simulink model "MotorMBD_TOP"  (R2018b)
settings: Solver=VariableStepAuto  StartTime=0.0  StopTime=1  RelTol=1e-3
values from neighbouring files (symbols this model uses):
  Jm = 0.0001    [parameter.m]
  Kdi = Ra*wc    (= 1002.79637503)    [parameter.m]
  Kdp = Ld*wc    (= 0.913156264643)    [parameter.m]
  Kqi = Ra*wc    (= 1002.79637503)    [parameter.m]
  Kqp = Lq*wc    (= 0.996932068739)    [parameter.m]
  Ksa = 3/Ksp    (= 35.8098621957)    [parameter.m]
  Ksi = Jm*wsc*(wsc/5)    (= 14.0367707038)    [parameter.m]
  Ksp = Jm*wsc    (= 0.0837758040957)    [parameter.m]
  Ld = 1.09e-4    (= 0.000109)    [parameter.m]
  Lq = 1.19e-4    (= 0.000119)    [parameter.m]
  Phia = 4.5e-3    (= 0.0045)    [parameter.m]
  Pn = 4    [parameter.m]
  Ra = 0.1197    [parameter.m]
  rpm2wrm = (2*pi)/60    (= 0.10471975512)    [parameter.m]
  taul = 0    [parameter.m]
  wrm2rpm = 60/(2*pi)    (= 9.54929658551)    [parameter.m]
settings Model: Creator=81803  LastModifiedBy=81803

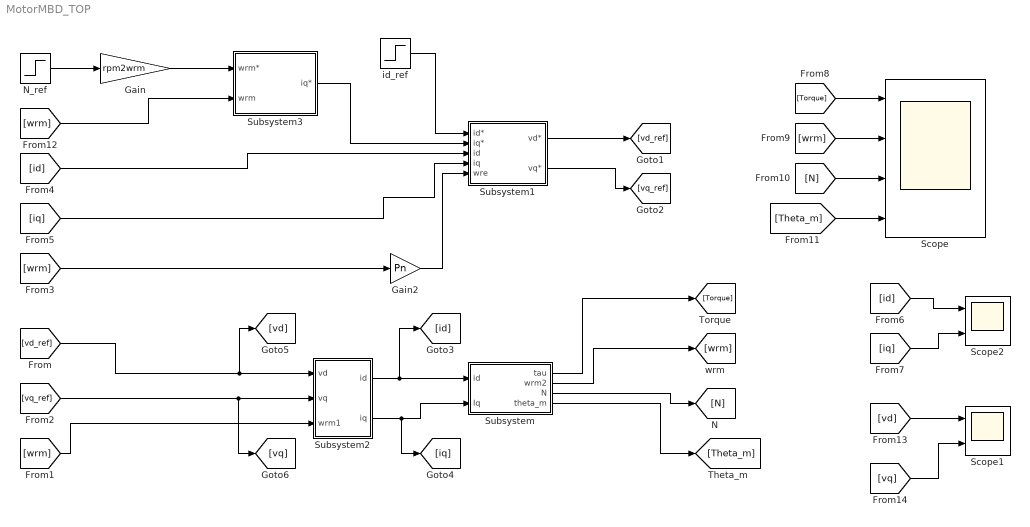
== system MotorMBD_TOP ==
  Gain : Gain  Gain=rpm2wrm
  Gain2 : Gain  Gain=Pn
  N_ref : Step  Time=0  After=3000  SampleTime=0
  Scope : Scope  NumInputPorts=4
  Scope1 : Scope  NumInputPorts=2
  Scope2 : Scope  NumInputPorts=2
  Subsystem : Subsystem
  Subsystem1 : Subsystem
  Subsystem2 : Subsystem
  Subsystem3 : Subsystem
  id_ref : Step  Time=0  After=0  SampleTime=0
  wires:
  id_ref/1 -> Subsystem1/1(id*)
  Subsystem3/1(iq*) -> Subsystem1/2(iq*)
  [id] -> Subsystem1/3(id)
  [iq] -> Subsystem1/4(iq)
  [wrm] -> Gain2/1
  Subsystem1/1(vd*) -> [vd_ref]
  Subsystem1/2(vq*) -> [vq_ref]
  [vd_ref] -> [vd], Subsystem2/1(vd)
  Subsystem2/1(id) -> [id], Subsystem/1(id)
  [vq_ref] -> [vq], Subsystem2/2(vq)
  Subsystem2/2(iq) -> [iq], Subsystem/2(Iq)
  Subsystem/1(tau) -> [Torque]
  [wrm] -> Subsystem2/3(wrm1)
  Subsystem/4(theta_m) -> [Theta_m]
  Subsystem/2(wrm2) -> [wrm]
  Subsystem/3(N) -> [N]
  [id] -> Scope2/1
  [iq] -> Scope2/2
  [Torque] -> Scope/1
  [wrm] -> Scope/2
  [N] -> Scope/3
  [Theta_m] -> Scope/4
  Gain/1 -> Subsystem3/1(wrm*)
  [wrm] -> Subsystem3/2(wrm)
  N_ref/1 -> Gain/1
  Gain2/1 -> Subsystem1/5(wre)
  [vd] -> Scope1/1
  [vq] -> Scope1/2

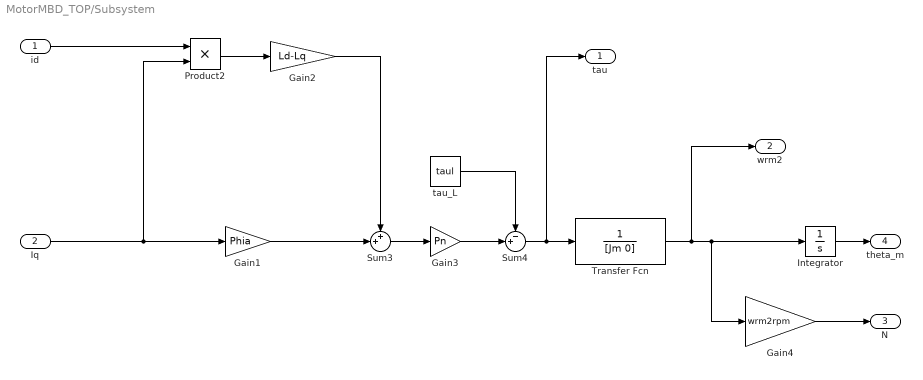
== system MotorMBD_TOP/Subsystem ==
  id : Inport
  Iq : Inport  Port=2
  Gain1 : Gain  Gain=Phia
  Gain2 : Gain  Gain=Ld-Lq
  Gain3 : Gain  Gain=Pn
  Gain4 : Gain  Gain=wrm2rpm
  Integrator : Integrator
  Product2 : Product
  Sum3 : Sum  Inputs=++|
  Sum4 : Sum  Inputs=-+|
  Transfer Fcn : TransferFcn  Denominator=[Jm 0]
  tau_L : Constant  Value=taul
  tau : Outport
  wrm2 : Outport  Port=2
  N : Outport  Port=3
  theta_m : Outport  Port=4
  wires:
  Product2/1 -> Gain2/1
  Sum3/1 -> Gain3/1
  Gain2/1 -> Sum3/1
  Iq/1 -> Product2/2, Gain1/1
  id/1 -> Product2/1
  Gain1/1 -> Sum3/2
  Transfer Fcn/1 -> wrm2/1, Gain4/1, Integrator/1
  Sum4/1 -> tau/1, Transfer Fcn/1
  Gain3/1 -> Sum4/2
  tau_L/1 -> Sum4/1
  Integrator/1 -> theta_m/1
  Gain4/1 -> N/1

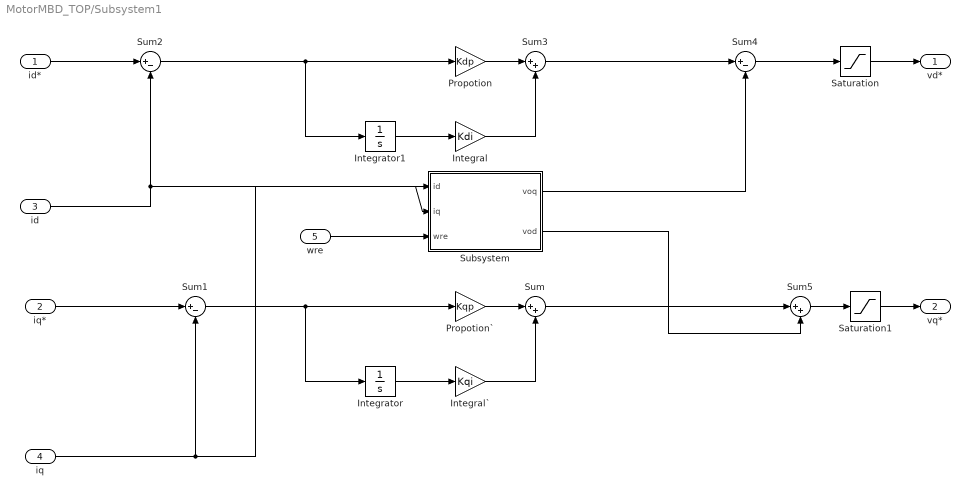
== system MotorMBD_TOP/Subsystem1 ==
  id* : Inport
  iq* : Inport  Port=2
  id : Inport  Port=3
  iq : Inport  Port=4
  wre : Inport  Port=5
  Integral : Gain  Gain=Kdi
  Integral` : Gain  Gain=Kqi
  Integrator : Integrator
  Integrator1 : Integrator
  Propotion : Gain  Gain=Kdp
  Propotion` : Gain  Gain=Kqp
  Saturation : Saturate  UpperLimit=7.32  LowerLimit=-7.32
  Saturation1 : Saturate  UpperLimit=7.32  LowerLimit=-7.32
  Subsystem : Subsystem
  Sum : Sum  Inputs=|++
  Sum1 : Sum  Inputs=|+-
  Sum2 : Sum  Inputs=|+-
  Sum3 : Sum  Inputs=|++
  Sum4 : Sum  Inputs=|+-
  Sum5 : Sum  Inputs=|++
  vd* : Outport
  vq* : Outport  Port=2
  wires:
  iq*/1 -> Sum1/1
  Propotion`/1 -> Sum/1
  Integrator/1 -> Integral`/1
  Propotion/1 -> Sum3/1
  Integral/1 -> Sum3/2
  wre/1 -> Subsystem/3(wre)
  Sum4/1 -> Saturation/1
  Sum/1 -> Sum5/1
  id/1 -> Subsystem/2(iq), Sum2/2
  Sum5/1 -> Saturation1/1
  id*/1 -> Sum2/1
  Sum2/1 -> Integrator1/1, Propotion/1
  Integral`/1 -> Sum/2
  Subsystem/2(vod) -> Sum5/2
  Sum1/1 -> Integrator/1, Propotion`/1
  iq/1 -> Subsystem/1(id), Sum1/2
  Subsystem/1(voq) -> Sum4/2
  Sum3/1 -> Sum4/1
  Integrator1/1 -> Integral/1
  Saturation1/1 -> vq*/1
  Saturation/1 -> vd*/1

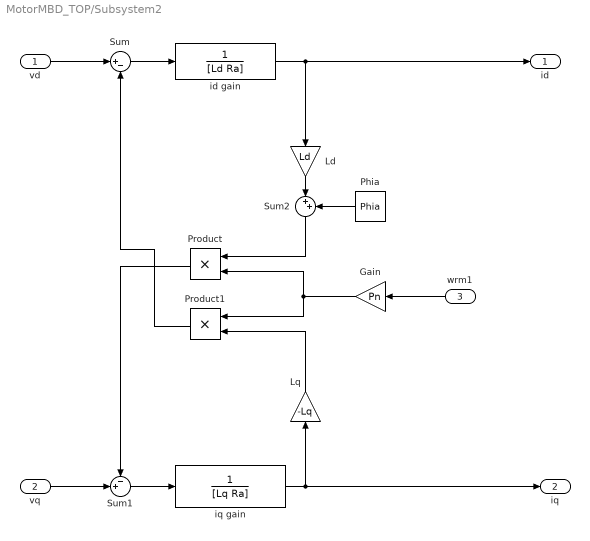
== system MotorMBD_TOP/Subsystem2 ==
  vd : Inport
  vq : Inport  Port=2
  wrm1 : Inport  Port=3
  Gain : Gain  Gain=Pn
  Ld : Gain  Gain=Ld
  Lq : Gain  Gain=-Lq
  Phia : Constant  Value=Phia
  Product : Product
  Product1 : Product
  Sum : Sum  Inputs=|+-
  Sum1 : Sum  Inputs=-+|
  Sum2 : Sum  Inputs=|++
  id gain : TransferFcn  Denominator=[Ld Ra]
  iq gain : TransferFcn  Denominator=[Lq Ra]
  id : Outport
  iq : Outport  Port=2
  wires:
  Gain/1 -> Product1/1, Product/2
  Phia/1 -> Sum2/2
  Sum1/1 -> iq gain/1
  Product/1 -> Sum1/1
  Sum2/1 -> Product/1
  id gain/1 -> id/1, Ld/1
  Product1/1 -> Sum/2
  Lq/1 -> Product1/2
  iq gain/1 -> Lq/1, iq/1
  wrm1/1 -> Gain/1
  vd/1 -> Sum/1
  Ld/1 -> Sum2/1
  Sum/1 -> id gain/1
  vq/1 -> Sum1/2

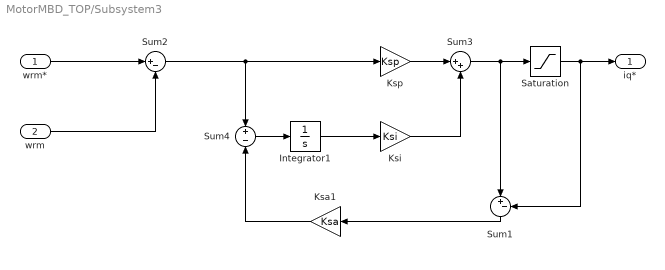
== system MotorMBD_TOP/Subsystem3 ==
  wrm* : Inport
  wrm : Inport  Port=2
  Integrator1 : Integrator
  Ksa1 : Gain  Gain=Ksa
  Ksi : Gain  Gain=Ksi
  Ksp : Gain  Gain=Ksp
  Saturation : Saturate  UpperLimit=25  LowerLimit=-25
  Sum1 : Sum  Inputs=|+-
  Sum2 : Sum  Inputs=|+-
  Sum3 : Sum  Inputs=|++
  Sum4 : Sum  Inputs=+-
  iq* : Outport
  wires:
  Sum2/1 -> Ksp/1, Sum4/1
  Integrator1/1 -> Ksi/1
  Sum3/1 -> Sum1/1, Saturation/1
  Ksp/1 -> Sum3/1
  wrm/1 -> Sum2/2
  Ksi/1 -> Sum3/2
  wrm*/1 -> Sum2/1
  Saturation/1 -> Sum1/2, iq*/1
  Sum1/1 -> Ksa1/1
  Sum4/1 -> Integrator1/1
  Ksa1/1 -> Sum4/2

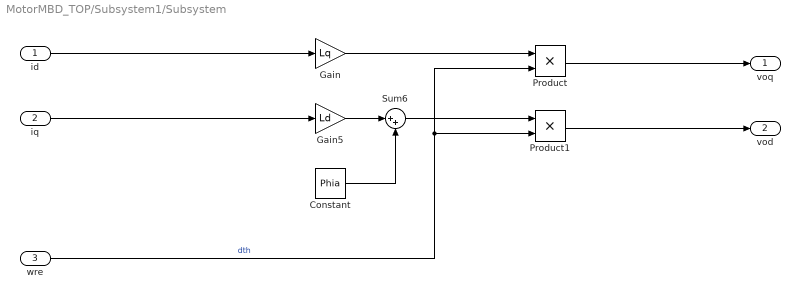
== system MotorMBD_TOP/Subsystem1/Subsystem ==
  id : Inport
  iq : Inport  Port=2
  wre : Inport  Port=3
  Constant : Constant  Value=Phia
  Gain : Gain  Gain=Lq
  Gain5 : Gain  Gain=Ld
  Product : Product
  Product1 : Product
  Sum6 : Sum  Inputs=|++
  voq : Outport
  vod : Outport  Port=2
  wires:
  Sum6/1 -> Product1/1
  Constant/1 -> Sum6/2
  Gain/1 -> Product/1
  wre/1 -> Product/2, Product1/2  "dth"
  Gain5/1 -> Sum6/1
  Product/1 -> voq/1
  iq/1 -> Gain5/1
  Product1/1 -> vod/1
  id/1 -> Gain/1
